simulink model "a_ASXX_MWIN_FLW_filupxxxxg_A"  (R2016b)
settings: Solver=FixedStepDiscrete  StartTime=0.0  StopTime=1  RelTol=1e-3  EnableMultiTasking=on
values from neighbouring files (symbols this model uses):
  Cbx_cyl_fill_efy_intk_mfld_prs_atm_prs_cor_cho = true    [Calib_mdl_RSA.m]
  Cbx_cyl_fill_efy_opt_cho = false    [Calib_mdl_RSA.m]
  Cbx_cyl_fill_igr_opt_cho = false    [Calib_mdl_RSA.m]
  Cnx_cyl_fill_ex_mfld_prs_cor_cho = 0    [Cal_basic.m]
  Cnx_cyl_nr_conf = 3    [Cal_basic.m]
  Cxx_cyl_fill_efy_drv_max = 20    [Calib_mdl_RSA.m]
  Cxx_cyl_fill_efy_dyn_max = 0.15    [Calib_mdl_RSA.m]
  Cxx_cyl_fill_efy_dyn_min = 0    [Calib_mdl_RSA.m]
  Cxx_cyl_fill_efy_dz = 0.45    [Calib_mdl_RSA.m]
  Cxx_cyl_fill_efy_vvt_ofs = 0    [Calib_mdl_RSA.m]
  Cxx_cyl_fill_trap_area_h_thd = 0.2    [Cal_basic.m]
  Cxx_cyl_fill_trap_area_l_thd = 0.1    [Cal_basic.m]
  Cxx_cyl_fill_trap_efy_dz_l_thd = 1    [Cal_basic.m]
  Cxx_cyl_fill_trap_efy_dz_neg_slop = -0.5    [Cal_basic.m]
  Cxx_cyl_fill_trap_efy_dz_pos_slop = 0.5    [Cal_basic.m]
  Cxx_cyl_vol = 3.9961e-04*3    (= 0.00119883)    [Cal_basic.m]    (also in Calib_mdl_RSA.m = 0.00119900004938)
  Cxx_min_cyl_fill_mdl_ex_mfld_prs_rat_cor = 0    [Cal_basic.m]
  Nnx_eng_run_stt = 2    [Calib_mdl_RSA.m]
  Nxx_atm_kpa = 101.3    [Cal_basic.m]
  Nxx_k_degc = 273.15    [Cal_basic.m]
  Nxx_kilo_bas = 1000    [Cal_basic.m]
  Nxx_wht_pgc_j_kg = 287    [Cal_basic.m]
undefined symbols (not defined in the file or in its folder): docblock
libraries: AEMS_Standard_Library x63, simulink x1
(part 1 of 3)
Description:
  | TITLE: Calculation of the volumetric efficiency correction
  | Object of the element: This document specifies the calculation of the cylinder fill-up efficiency depending on pressure, engine speed,VVT angle and VVL position.
settings Model: Creator=z005139  LastModifiedBy=a002701
settings Model: ModifiedHistory=|
  | <Delivery_cycle>: MD13
  | <Author>: f046779
  | <Revision>: 7-0
  | <Nature_of_modifications>: <IS130624>: AEMS / EAL computational problem during a smooth start HR12DDV
  | <Nature_of_modifications>: <IS130784>: AEMS / Wrong calculation of trapping efficiency
  | <Nature_of_modifications>: <IS130844>: AEMS / Insufficient air filling correction in altitude
  | 
  | <Delivery_cycle>: MD12
  | <Author>: p080490
  | <Revision>: 6-0
  | <Nature_of_modifications>: <IS129656>: AEMS / Estimated trapping efficiency impact on exhaust richness setpoint
  | 
  | <Delivery_cycle>: MD11
  | <Author>: p097653
  | <Revision>: 5-0
  | <Nature_of_modifications>: <CR010224>: [IS][AEMS Step2] Issue correction for AE MD11 modules
  | <Nature_of_modifications>: <CR009896>: [AEMS Step2][LPG][Archi] Legacy Migration pour MD11
  | <Nature_of_modifications>: <IS128079>: AEMS / Wrong air filling model correction with atmospheric pressure and deltaP_GPF
  | 
  | <Delivery_cycle>: MD10
  | <Author>: a002701
  | <Revision>: 4-0
  | <Nature_of_modifications>: <CR009236>: [AEMS Step1.9][Gasoline] Update of Engine model improvement (part2)
  | 
  | <Delivery_cycle>: MD09
  | <Author>: p095922
  | <Revision>: 3-0
  | <Nature_of_modifications>: <CR009534>: [IS][A-EMS] Issue correction for AE MD09 modules
  | <Nature_of_modifications>: <IS124783>: AEMS /Wrong constant (Nxx_atm_hpa) used for atmospheric pressure (kpa) related calculation
  | <Nature_of_modifications>: <IS124785>: AEMS /Wrong IGR mass caculation of air filling model
  | 
  | <Delivery_cycle>: MD08
  | <Author>: a002701
  | <Revision>: 2-0
  | <Nature_of_modifications>: <CR006368> : [A-ems step2]  [EFE] Engine model improvement
  | <Nature_of_modifications>: <CR006372>: VVT drift learning usage
  | 
  | <Delivery_cycle>: MD07.02
  | <Author>: p095922
  | <Revision>: 1-0
  | <Nature_of_modifications>: <CR006362>: [A-ems step2] [SUPAS] Intake manifold & boost pressure setpoint
  | <Nature_of_modifications>: <CR008239>: Engine filling & Air flow sensor management
  | <Nature_of_modifications>: <IS122176>: AEMS /[MDL] Underflow occurs for the Output variable Vxx_fill_efv_fuel_rat_raw_20ms
  | 
  | <Delivery_cycle>: MD06.02
  | <Author>: p092015
  | <Revision>: 0-0
  | <Nature_of_modifications>: <CR007978>: [AEMS Step1.9] [Gasoline] GE-R migration
  | 
  | <Delivery_cycle>: LM55_01
  | <Author>: Vuong-son LUONG
  | <Revision>: Rev 35.0
  | <Nature_of_modifications>: <CR007978>: [AEMS Step1.9] [Gasoline] GE-R migration (DMFI04672: [WAMA]: Needed dictionary update for LM55)
  | 
  | <Delivery_cycle>: LM52_01
  | <Author>: Rodolphe BOU TAYEH
  | <Revision>: Rev 34.0
  | <Nature_of_modifications>: <CR007978>: [AEMS Step1.9] [Gasoline] GE-R migration (DMFI04008[LPG] New labels for a specific LPG tuning - Torque management)
  | 
  | <Delivery_cycle>: LM50_01
  | <Author>: Bada NDOYE
  | <Revision>: Rev 33.0
  | <Nature_of_modifications>: <CR007978>: [AEMS Step1.9] [Gasoline] GE-R migration (DMFI03942: [MXAM] : MXAM rules update for LM50)
  | <Nature_of_modifications>: <CR007978>: [AEMS Step1.9] [Gasoline] GE-R migration (DMFI03944 [Tool] Models conversion into slx format for LM50)
  | 
  | <Delivery_cycle>: LM49
  | <Author>: Sarah TALEB
  | <Revision>: Rev 32.0
  | <Nature_of_modifications>: <CR007978>: [AEMS Step1.9] [Gasoline] GE-R migration (DMFI03797 [FLEX] Fill-up correction during transient conditions in Flex Fuel applications)
  | 
  | <Delivery_cycle>: LM47_01
  | <Author>: R.IRAQI
  | <Revision>: Rev 31.0
  | <Nature_of_modifications>: <CR007978>: [AEMS Step1.9] [Gasoline] GE-R migration (DMFI03552 [MXAM] : MXAM rules update for LM47)
  | <Nature_of_modifications>: <CR007978>: [AEMS Step1.9] [Gasoline] GE-R migration (DMFI03553: [WAMA]: Needed dictionary update for LM47)
  | 
  | <Delivery_cycle>: LM42_01
  | <Author>: Hugo DAMANCE
  | <Revision>: Rev 30.0
  | <Nature_of_modifications>: <CR007978>: [AEMS Step1.9] [Gasoline] GE-R migration (DMFI02878 [MXAM] : MXAM rules update for LM42)
  | 
  | <Delivery_cycle>: LM41_01
  | <Author>: Antoine NAIIM HABIB
  | <Revision>: Rev 29.0
  | <Nature_of_modifications>: <CR007978>: [AEMS Step1.9] [Gasoline] GE-R migration (ISMET27009 K3: [SPEC] Wrong use of Interp library with shared axis in IN_ASI_IAF_2)
  | <Nature_of_modifications>: <CR007978>: [AEMS Step1.9] [Gasoline] GE-R migration (DMFI02746: [Floating] Actual integer data typing to reach one click auto-coding)
  | <Nature_of_modifications>: <CR007978>: [AEMS Step1.9] [Gasoline] GE-R migration (ISMET29395 K4: [SPEC] Evolution of range for coherency in a_in_asi_iaf_filupxx_xxx_xx_g_a)
  | 
  | <Delivery_cycle>: AEG_39_01
  | <Author>: Cheng-Qiang HE
  | <Revision>: Rev 28.0
  | <Nature_of_modifications>: <CR007978>: [AEMS Step1.9] [Gasoline] GE-R migration (ISSUP21633 K3: Issue in model La table Ctp_fill_efy_cor_dyn_amp_rat ne doit pas avoir d'axes partages)
  | <Nature_of_modifications>: <CR007978>: [AEMS Step1.9] [Gasoline] GE-R migration (DMFI02368: [Floating] Modification of specification to comply with floating autocoding LM39)
  | 
  | <Delivery_cycle>: AEG_34_01
  | <Author>: YOBOUE Konan
  | <Revision>: Rev 27.0
  | <Nature_of_modifications>: <CR007978>: [AEMS Step1.9] [Gasoline] GE-R migration (IS19506 (K2): Ctb_mat2 is not anymore referenced by InAsiIat)
  | 
  | <Delivery_cycle>: LM_XX
  | <Author>: KIEFFER Steve
  | <Revision>: Rev 26.0
  | <Nature_of_modifications>: <CR007978>: [AEMS Step1.9] [Gasoline] GE-R migration (ISMAP18189 : Altitude correction for fill-up model)
  | 
  | <Delivery_cycle>: LM_XX
  | <Author>: KIEFFER Steve
  | <Revision>: Rev 25.0
  | <Nature_of_modifications>: <CR007978>: [AEMS Step1.9] [Gasoline] GE-R migration (ISSUP K2 13588 : Breakpoints shall be given under referenced section in MID)
  | <Nature_of_modifications>: <CR007978>: [AEMS Step1.9] [Gasoline] GE-R migration (ISMAP K3 15074 : Range correction of cmp_n_map_fill_efv_ofs_alco)
  | 
  | <Delivery_cycle>: LM_XX
  | <Author>: THOUVENEL Nicolas
  | <Revision>: Rev 24.0
  | <Nature_of_modifications>: <CR007978>: [AEMS Step1.9] [Gasoline] GE-R migration (ISMET13261 : Modification for dynamic fill-up efficiency computation)
  | 
  | <Delivery_cycle>: LM_XX
  | <Author>: THOUVENEL Nicolas
  | <Revision>: Rev 23.0
  | <Nature_of_modifications>: <CR007978>: [AEMS Step1.9] [Gasoline] GE-R migration (ISMAP 11648 : Dynamic Over fill-up)
  | <Nature_of_modifications>: <CR007978>: [AEMS Step1.9] [Gasoline] GE-R migration (ISMET 12293 : Taking into account of injected fuel flow drift function as Tcarb over F4Rt87x)
  | <Nature_of_modifications>: <CR007978>: [AEMS Step1.9] [Gasoline] GE-R migration (ISMET 12394 : Dictionary to be modified for dissociating variables Vxx_fill_efy_cor_dyn_amp_raw &amp; Vxx_fill_efy_cor_dyn_raw)
  | <Nature_of_modifications>: <CR007978>: [AEMS Step1.9] [Gasoline] GE-R migration (ISMAP 12637 : Basic tuning impossible with ASG_26 (implementation of cylinder deactivation)
  | <Nature_of_modifications>: <CR007978>: [AEMS Step1.9] [Gasoline] GE-R migration (ISMET 12912 : Modification of logical naming for cartography of cylinder deactivation)
  | 
  | <Delivery_cycle>: LM_XX
  | <Author>: BANZET Sebastien
  | <Revision>: Rev 22.0
  | <Nature_of_modifications>: <CR007978>: [AEMS Step1.9] [Gasoline] GE-R migration (DMFI Amont 207 : Cylinder deactivation)
  | <Nature_of_modifications>: <CR007978>: [AEMS Step1.9] [Gasoline] GE-R migration (DMFI 833 : [Flex/Gasoline] : Separated management for Flex &amp; Gasoline tuning values #2)
  | <Nature_of_modifications>: <CR007978>: [AEMS Step1.9] [Gasoline] GE-R migration (ISMET 10136 : implementation of intermediate variables for fill-up efficiency calculation)
  | <Nature_of_modifications>: <CR007978>: [AEMS Step1.9] [Gasoline] GE-R migration (ISMET 10468 : Check revision of timer block)
  | 
  | <Delivery_cycle>: LM_XX
  | <Author>: THOUVENEL Nicolas
  | <Revision>: Rev 21.0
  | <Nature_of_modifications>: <CR007978>: [AEMS Step1.9] [Gasoline] GE-R migration (ISMET 09504 : Fill-up and Trapping models correction with taking into account atmospheric pressure)
  | 
  | <Delivery_cycle>: LM_XX
  | <Author>: HEBERT
  | <Revision>: Rev 20.0
  | <Nature_of_modifications>: <CR007978>: [AEMS Step1.9] [Gasoline] GE-R migration (ISMET05853: Modification of Vxx_vvt_fill_efv_cor_fac1 range and resol. Correction of Cmp_vvt_fill_efv_cor_fac1 bounds) (a_in_asi_iaf_filupxx_xxx_xx_g_a)
  | 
  | <Delivery_cycle>: LM_XX
  | <Author>: THOUVENEL
  | <Revision>: Rev 19.3
  | <Nature_of_modifications>: <CR007978>: [AEMS Step1.9] [Gasoline] GE-R migration (Update to ISMET 05742) (a_in_asi_iaf_filupxx_xxx_xx_g_a)
  | 
  | <Delivery_cycle>: LM_XX
  | <Author>: THOUVENEL
  | <Revision>: Rev 19.2
  | <Nature_of_modifications>: <CR007978>: [AEMS Step1.9] [Gasoline] GE-R migration (Correction of resolution of Vxx_fill_efy_cor_dyn) (a_in_asi_iaf_filupxx_xxx_xx_g_a)
  | 
  | <Delivery_cycle>: LM_XX
  | <Author>: THOUVENEL
  | <Revision>: Rev 19.1
  | <Nature_of_modifications>: <CR007978>: [AEMS Step1.9] [Gasoline] GE-R migration (IS 04502 : "Missing documentation in a_in_asi_iaf_filupxx_xxx_xx_g_a(19.0)") (a_in_asi_iaf_filupxx_xxx_xx_g_a)
  | 
  | <Delivery_cycle>: LM_XX
  | <Author>: THOUVENEL
  | <Revision>: Rev 19.0
  | <Nature_of_modifications>: <CR007978>: [AEMS Step1.9] [Gasoline] GE-R migration (Implementation of volumetric correction for Dual VVT (intake, exhaust)) (a_in_asi_iaf_filupxx_xxx_xx_g_a)
  | 
  | <Delivery_cycle>: LM_XX
  | <Author>: LENOIR
  | <Revision>: Rev 18.0
  | <Nature_of_modifications>: <CR007978>: [AEMS Step1.9] [Gasoline] GE-R migration (ISMAP_2163: Add New calibration Cmp_n_map_cor_dyn_amp, Ctp_fill_efy_cor_dyn_amp_rat, Ctb_fill_efy_cor_dyn_amp, New Input Vxx_amp, Change resolution of Cmp_n_map_cor_dyn_th) (a_in_asi_iaf_filupxx_xxx_xx_g_a)
  | 
  | <Delivery_cycle>: LM_XX
  | <Author>: LENOIR
  | <Revision>: Rev 17.0
  | <Nature_of_modifications>: <CR007978>: [AEMS Step1.9] [Gasoline] GE-R migration (IS_MAP 420 :  Add the "thermic" factor to correct the fill-up efficiency (figure 4) =&gt; New Inputs : Vsx_eng, Vxx_tco=&gt; New internal variables :Vxx_fill_efy_cor_dyn, Vxx_fill_efy_cor_dyn_raw.=&gt; New calibrations : Cmp_n_map_cor_dyn_th, Ctb_n_fill_efy_cor_dyn, Ctb_tco2, Ctp_map_n_ftc,  Cxx_fill_efy_cor_dyn_max, Cxx_fill_efy_cor_dyn_min,  Nsx_eng_aut) (a_in_asi_iaf_filupxx_xxx_xx_g_a)
  | 
  | <Delivery_cycle>: LM_XX
  | <Author>: WALRAVE
  | <Revision>: Rev 16.0
  | <Nature_of_modifications>: <CR007978>: [AEMS Step1.9] [Gasoline] GE-R migration (reopening of ISMAP 32 : Resolutions of Cmp_vvt_fill_efv_cor_fac1, Cmp_vvt_fill_efv_cor_fac2, Vxx_vvt_fill_efv_cor_fac1, Vxx_vvt_fill_efv_cor_fac2 has been divided by 256. ranges unchanged) (a_in_asi_iaf_filupxx_xxx_xx_g_a)
  | 
  | <Delivery_cycle>: LM_XX
  | <Author>: WALRAVE
  | <Revision>: Rev 15.0
  | <Nature_of_modifications>: <CR007978>: [AEMS Step1.9] [Gasoline] GE-R migration (Alcool settings added offset of fill up efficiency coming form alcoxxx spec as well as specific temperature correction for alcool LPG removed new document model) (a_in_asi_iaf_filupxx_xxx_xx_g_a)
  | 
  | <Delivery_cycle>: LM_XX
  | <Author>: WALRAVE
  | <Revision>: Rev 14.0
  | <Nature_of_modifications>: <CR007978>: [AEMS Step1.9] [Gasoline] GE-R migration (Bug correction on VVT parameter. Cmp_vvt_fill_efv_cor_fac1 and fac2 have a new resolution and range. As well as Vxx_vvt_fill_efv_cor_fac1 and fac2. Bloc names changed to respect rules) (a_in_asi_iaf_filupxx_xxx_xx_g_a)
  | 
  | <Delivery_cycle>: LM_XX
  | <Author>: ALLACH
  | <Revision>: Rev 13.0
  | <Nature_of_modifications>: <CR007978>: [AEMS Step1.9] [Gasoline] GE-R migration (Add Shared index Vxb_n in Cmp_vvt_fill_efv_cor_fac1 Cmp_vvt_fill_efv_cor_fac2 Cmp_n_map_fill_efv Cmp_n_map_fill_efv_lpg RSA_BKPT_2D block) (a_in_asi_iaf_filupxx_xxx_xx_g_a)
  | 
  | <Delivery_cycle>: LM_XX
  | <Author>: WALRAVE
  | <Revision>: Rev 12.0
  | <Nature_of_modifications>: <CR007978>: [AEMS Step1.9] [Gasoline] GE-R migration (Engine speed IVLD removed. VVT IVLD removed. Slew rate is now before the deadzone on filtered fill-up efficiency. Comments corrected) (a_in_asi_iaf_filupxx_xxx_xx_g_a)
  | 
  | <Delivery_cycle>: LM_XX
  | <Author>: WALRAVE
  | <Revision>: Rev 11.0
  | <Nature_of_modifications>: <CR007978>: [AEMS Step1.9] [Gasoline] GE-R migration (Update of the IVLD construction. Added init values. Removed replacement values for inputs Document model modified) (a_in_asi_iaf_filupxx_xxx_xx_g_a)
  | 
  | <Delivery_cycle>: LM_XX
  | <Author>: WALRAVE
  | <Revision>: Rev 10.0
  | <Nature_of_modifications>: <CR007978>: [AEMS Step1.9] [Gasoline] GE-R migration (Modification for IS 109 : Library blocks are used instead in the filter block for the throttle command) (a_in_asi_iaf_filupxx_xxx_xx_g_a)
  | 
  | <Delivery_cycle>: LM_XX
  | <Author>: WALRAVE
  | <Revision>: Rev 9.0
  | <Nature_of_modifications>: <CR007978>: [AEMS Step1.9] [Gasoline] GE-R migration (strategy for ON/OFF VVT removed. Vbx_vvt_cart_ti removed) (a_in_asi_iaf_filupxx_xxx_xx_g_a)
  | 
  | <Delivery_cycle>: LM_XX
  | <Author>: WALRAVE
  | <Revision>: Rev 8.0
  | <Nature_of_modifications>: <CR007978>: [AEMS Step1.9] [Gasoline] GE-R migration (Coherency done. vvt variables changed into standard types) (a_in_asi_iaf_filupxx_xxx_xx_g_a)
  | 
  | <Delivery_cycle>: LM_XX
  | <Author>: WALRAVE
  | <Revision>: Rev 7.0
  | <Nature_of_modifications>: <CR007978>: [AEMS Step1.9] [Gasoline] GE-R migration (New output Vxx_eng_vol_fill_efy_fil created for throttle command. Deadzone filter + rate limiter) (a_in_asi_iaf_filupxx_xxx_xx_g_a)
  | 
  | <Delivery_cycle>: LM_XX
  | <Author>: WALRAVE
  | <Revision>: Rev 6.0
  | <Nature_of_modifications>: <CR007978>: [AEMS Step1.9] [Gasoline] GE-R migration (RSI on RD8_020: Vxx_vvt_fill_efv_cor_fac2 range, resol and unit modified. Cmp_vvt_fill_efv_cor_fac2 range, resol &amp; unit modified. Several units corrected to be more explicit and standard) (a_in_asi_iaf_filupxx_xxx_xx_g_a)
  | 
  | <Delivery_cycle>: LM_XX
  | <Author>: PORCHEROT
  | <Revision>: Rev 5.0
  | <Nature_of_modifications>: <CR007978>: [AEMS Step1.9] [Gasoline] GE-R migration (Comment and state changed for Vsx_n_vld) (a_in_asi_iaf_filupxx_xxx_xx_g_a)
  | 
  | <Delivery_cycle>: LM_XX
  | <Author>: WALRAVE
  | <Revision>: Rev 4.0
  | <Nature_of_modifications>: <CR007978>: [AEMS Step1.9] [Gasoline] GE-R migration (Bloc "Validity_indicator" modified (two NOT added). Correction of Ctb_mat2 (input variable)) (a_in_asi_iaf_filupxx_xxx_xx_g_a)
  | 
  | <Delivery_cycle>: LM_XX
  | <Author>: WALRAVE
  | <Revision>: Rev 3.0
  | <Nature_of_modifications>: <CR007978>: [AEMS Step1.9] [Gasoline] GE-R migration (Validity indicators added. Correction for RSI 63 : resolution of Cmp_vvt_fill_efv_cor_fac1 modified) (a_in_asi_iaf_filupxx_xxx_xx_g_a)
  | 
  | <Delivery_cycle>: LM_XX
  | <Author>: ADMIN
  | <Revision>: Rev 2.1
  | <Nature_of_modifications>: <CR007978>: [AEMS Step1.9] [Gasoline] GE-R migration (Ctb_prs ( New max = 20000]), Vxx_in_vvtc_angl ( New max = 96[ New unit = DegCrk), Vxx_map ( New max = 20000])) (a_in_asi_iaf_filupxx_xxx_xx_g_a)
  | 
  | <Delivery_cycle>: LM_XX
  | <Author>: WALRAVE
  | <Revision>: Rev 2.0
  | <Nature_of_modifications>: <CR007978>: [AEMS Step1.9] [Gasoline] GE-R migration (Dictionary update + cartography dimension changed) (a_in_asi_iaf_filupxx_xxx_xx_g_a)
  | 
  | <Delivery_cycle>: LM_XX
  | <Author>: WALRAVE
  | <Revision>: Rev 1.1
  | <Nature_of_modifications>: <CR007978>: [AEMS Step1.9] [Gasoline] GE-R migration (Range &amp; resol corrected) (a_in_asi_iaf_filupxx_xxx_xx_g_a)
  | 
  | <Delivery_cycle>: LM_XX
  | <Author>: WALRAVE
  | <Revision>: Rev 1.0
  | <Nature_of_modifications>: <CR007978>: [AEMS Step1.9] [Gasoline] GE-R migration (Fillup efficiency is now physical (ratio near 1).It includes the effect of temperature that was in a_im_airxx_a5_a) (a_in_asi_iaf_filupxx_xxx_xx_g_a)
settings DataIOCC: SaveFormat=StructureWithTime
settings OptimizationCC: DefaultUnderspecifiedDataType=single  LifeSpan=inf
settings DebuggingCC: SignalInfNanChecking=error  SignalRangeChecking=error  AlgebraicLoopMsg=error  ArtificialAlgebraicLoopMsg=error  SaveWithParameterizedLinksMsg=error  CheckSSInitialOutputMsg=off  BlockPriorityViolationMsg=error  MinStepSizeMsg=error  SolverPrmCheckMsg=warning  InheritedTsInSrcMsg=error  TasksWithSamePriorityMsg=error  SigSpecEnsureSampleTimeMsg=error  CheckMatrixSingularityMsg=error  IntegerOverflowMsg=error  ParameterUnderflowMsg=error  ParameterPrecisionLossMsg=none  ParameterTunabilityLossMsg=error  FixptConstUnderflowMsg=error  FixptConstOverflowMsg=error  FixptConstPrecisionLossMsg=error  UnderSpecifiedDataTypeMsg=warning  UnnecessaryDatatypeConvMsg=warning  SignalLabelMismatchMsg=warning  UnconnectedInputMsg=error  UnconnectedOutputMsg=error  UnconnectedLineMsg=error  SFcnCompatibilityMsg=error  FrameProcessingCompatibilityMsg=warning  BusObjectLabelMismatch=error  RootOutportRequireBusObject=error  AllowSymbolicDim=off  ModelReferenceIOMsg=warning  ModelReferenceIOMismatchMessage=error  UnknownTsInhSupMsg=error  ModelReferenceDataLoggingMessage=error  StateNameClashWarn=warning  SimStateInterfaceChecksumMismatchMsg=error  StrictBusMsg=ErrorOnBusTreatedAsVector  NonBusSignalsTreatedAsBus=error  SFUnusedDataAndEventsDiag=error  SFInvalidInputDataAccessInChartInitDiag=error  SFTransitionOutsideNaturalParentDiag=error  SFUnreachableExecutionPathDiag=error  SFUndirectedBroadcastEventsDiag=error  SFOutputUsedAsStateInMooreChartDiag=none  SFTemporalDelaySmallerThanSampleTimeDiag=none  SFSelfTransitionDiag=error  SFExecutionAtInitializationDiag=none  UnitsInconsistencyMsg=none  AllowAutomaticUnitConversions=off
settings HardwareCC: ProdBitPerPointer=32  ProdBitPerSizeT=32  ProdBitPerPtrDiffT=32  ProdLargestAtomicInteger=Integer  ProdLargestAtomicFloat=None  ProdIntDivRoundTo=Undefined  ProdEndianess=Unspecified  ProdWordSize=32  ProdHWDeviceType=32-bit Generic
settings ModelReferenceCC: UpdateModelReferenceTargets=IfOutOfDate  EnableParallelModelReferenceBuilds=on  ParallelModelReferenceErrorOnInvalidPool=off  ModelReferenceNumInstancesAllowed=Single  PropagateSignalLabelsOutOfModel=off
settings SFSimCC: SFSimEcho=off  SimGenImportedTypeDefs=on
settings RTWCC: GenerateMakefile=off
settings GRTTargetCC: CodeReplacementLibrary=ANSI_C  MatFileLogging=off
settings ConfigComp: CovMetricSettings=dcmtrzoibsw  CovHtmlReporting=on  CovSaveCumulativeToWorkspaceVar=on  CovSaveSingleToWorkspaceVar=on  CovCumulativeReport=on

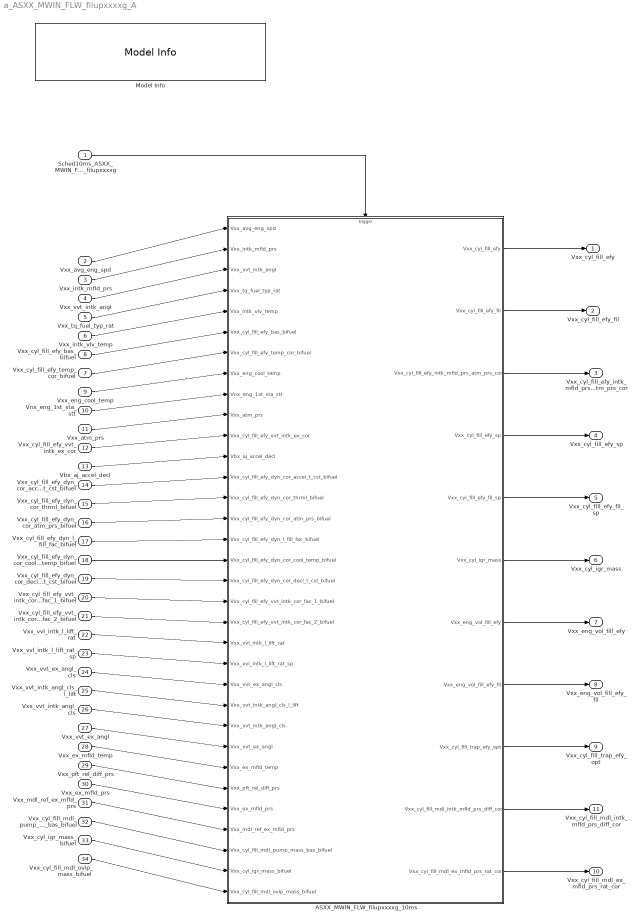
== system a_ASXX_MWIN_FLW_filupxxxxg_A ==
  Sched10ms_ASXX_MWIN_FLW_filupxxxxg : Inport  Interpolate=off  OutputFunctionCall=on
  Vxx_avg_eng_spd : Inport  Port=2  Interpolate=off
  Vxx_intk_mfld_prs : Inport  Port=3  Interpolate=off
  Vxx_vvt_intk_angl : Inport  Port=4  Interpolate=off
  Vxx_tq_fuel_typ_rat : Inport  Port=5  Interpolate=off
  Vxx_intk_vlv_temp : Inport  Port=6  Interpolate=off
  Vxx_cyl_fill_efy_temp_cor_bifuel : Inport  Port=7  Interpolate=off
  Vxx_cyl_fill_efy_bas_bifuel : Inport  Port=8  Interpolate=off
  Vxx_eng_cool_temp : Inport  Port=9  Interpolate=off
  Vnx_eng_1st_sta_stt : Inport  Port=10  Interpolate=off
  Vxx_atm_prs : Inport  Port=11  Interpolate=off
  Vxx_cyl_fill_efy_vvt_intk_ex_cor : Inport  Port=12  Interpolate=off
  Vbx_aj_accel_decl : Inport  Port=13  Interpolate=off
  Vxx_cyl_fill_efy_dyn_cor_accel_t_cst_bifuel : Inport  Port=14  Interpolate=off
  Vxx_cyl_fill_efy_dyn_cor_thrml_bifuel : Inport  Port=15  Interpolate=off
  Vxx_cyl_fill_efy_dyn_cor_atm_prs_bifuel : Inport  Port=16  Interpolate=off
  Vxx_cyl_fill_efy_dyn_l_fill_fac_bifuel : Inport  Port=17  Interpolate=off
  Vxx_cyl_fill_efy_dyn_cor_cool_temp_bifuel : Inport  Port=18  Interpolate=off
  Vxx_cyl_fill_efy_dyn_cor_decl_t_cst_bifuel : Inport  Port=19  Interpolate=off
  Vxx_cyl_fill_efy_vvt_intk_cor_fac_1_bifuel : Inport  Port=20  Interpolate=off
  Vxx_cyl_fill_efy_vvt_intk_cor_fac_2_bifuel : Inport  Port=21  Interpolate=off
  Vxx_vvl_intk_l_lift_rat : Inport  Port=22  Interpolate=off
  Vxx_vvl_intk_l_lift_rat_sp : Inport  Port=23  Interpolate=off
  Vxx_vvt_ex_angl_cls : Inport  Port=24  Interpolate=off
  Vxx_vvt_intk_angl_cls_l_lift : Inport  Port=25  Interpolate=off
  Vxx_vvt_intk_angl_cls : Inport  Port=26  Interpolate=off
  Vxx_vvt_ex_angl : Inport  Port=27  Interpolate=off
  Vxx_ex_mfld_temp : Inport  Port=28  Interpolate=off
  Vxx_pft_rel_diff_prs : Inport  Port=29  Interpolate=off
  Vxx_ex_mfld_prs : Inport  Port=30  Interpolate=off
  Vxx_mdl_ref_ex_mfld_prs : Inport  Port=31  Interpolate=off
  Vxx_cyl_fill_mdl_pump_mass_bas_bifuel : Inport  Port=32  Interpolate=off
  Vxx_cyl_igr_mass_bifuel : Inport  Port=33  Interpolate=off
  Vxx_cyl_fill_mdl_ovlp_mass_bifuel : Inport  Port=34  Interpolate=off
  ASXX_MWIN_FLW_filupxxxxg_10ms : Subsystem  Tag=[RUNNABLE]  TreatAsAtomicUnit=on  RTWFileName=InAsiIaf_Filupxx_xxxxxg
      settings: AttributesFormatString=%<Tag>  RTWSystemCode=Nonreusable function  RTWFcnNameOpts=Use subsystem name  RTWFileNameOpts=User specified
  Model Info : simulink/Model-Wide Utilities/Model Info  Frame=on  DisplayStringWithTags=|  HorizontalTextAlignment=Center  LeftAlignmentValue=0.5  SourceBlockDiagram=a_ASXX_MWIN_FLW_filupxxxxg_A  TagMaxNumber=20
      | Model Info
      | %<ModelVersion>
      | Editor: %<LastModifiedBy>
      | Last modified: %<LastModificationDate>
  Vxx_cyl_fill_efy : Outport
  Vxx_cyl_fill_efy_fil : Outport  Port=2
  Vxx_cyl_fill_efy_intk_mfld_prs_atm_prs_cor : Outport  Port=3
  Vxx_cyl_fill_efy_sp : Outport  Port=4
  Vxx_cyl_fill_efy_fil_sp : Outport  Port=5
  Vxx_cyl_igr_mass : Outport  Port=6
  Vxx_eng_vol_fill_efy : Outport  Port=7
  Vxx_eng_vol_fill_efy_fil : Outport  Port=8
  Vxx_cyl_fill_trap_efy_opt : Outport  Port=9
  Vxx_cyl_fill_mdl_ex_mfld_prs_rat_cor : Outport  Port=10
  Vxx_cyl_fill_mdl_intk_mfld_prs_diff_cor : Outport  Port=11
  wires:
  Vxx_cyl_fill_efy_vvt_intk_cor_fac_2_bifuel/1 -> ASXX_MWIN_FLW_filupxxxxg_10ms/20(Vxx_cyl_fill_efy_vvt_intk_cor_fac_2_bifuel)
  Vxx_cyl_fill_efy_vvt_intk_cor_fac_1_bifuel/1 -> ASXX_MWIN_FLW_filupxxxxg_10ms/19(Vxx_cyl_fill_efy_vvt_intk_cor_fac_1_bifuel)
  Vxx_cyl_fill_efy_dyn_cor_decl_t_cst_bifuel/1 -> ASXX_MWIN_FLW_filupxxxxg_10ms/18(Vxx_cyl_fill_efy_dyn_cor_decl_t_cst_bifuel)
  Vxx_cyl_fill_efy_dyn_cor_cool_temp_bifuel/1 -> ASXX_MWIN_FLW_filupxxxxg_10ms/17(Vxx_cyl_fill_efy_dyn_cor_cool_temp_bifuel)
  Vxx_cyl_fill_efy_dyn_l_fill_fac_bifuel/1 -> ASXX_MWIN_FLW_filupxxxxg_10ms/16(Vxx_cyl_fill_efy_dyn_l_fill_fac_bifuel)
  Vxx_cyl_fill_efy_dyn_cor_atm_prs_bifuel/1 -> ASXX_MWIN_FLW_filupxxxxg_10ms/15(Vxx_cyl_fill_efy_dyn_cor_atm_prs_bifuel)
  Vxx_cyl_fill_efy_dyn_cor_thrml_bifuel/1 -> ASXX_MWIN_FLW_filupxxxxg_10ms/14(Vxx_cyl_fill_efy_dyn_cor_thrml_bifuel)
  Vxx_cyl_fill_efy_dyn_cor_accel_t_cst_bifuel/1 -> ASXX_MWIN_FLW_filupxxxxg_10ms/13(Vxx_cyl_fill_efy_dyn_cor_accel_t_cst_bifuel)
  Vxx_avg_eng_spd/1 -> ASXX_MWIN_FLW_filupxxxxg_10ms/1(Vxx_avg_eng_spd)
  Vxx_intk_mfld_prs/1 -> ASXX_MWIN_FLW_filupxxxxg_10ms/2(Vxx_intk_mfld_prs)
  Vxx_vvt_intk_angl/1 -> ASXX_MWIN_FLW_filupxxxxg_10ms/3(Vxx_vvt_intk_angl)
  Vxx_tq_fuel_typ_rat/1 -> ASXX_MWIN_FLW_filupxxxxg_10ms/4(Vxx_tq_fuel_typ_rat)
  Vxx_intk_vlv_temp/1 -> ASXX_MWIN_FLW_filupxxxxg_10ms/5(Vxx_intk_vlv_temp)
  Sched10ms_ASXX_MWIN_FLW_filupxxxxg/1 -> ASXX_MWIN_FLW_filupxxxxg_10ms/Trigger
  Vxx_cyl_fill_efy_temp_cor_bifuel/1 -> ASXX_MWIN_FLW_filupxxxxg_10ms/7(Vxx_cyl_fill_efy_temp_cor_bifuel)
  Vxx_cyl_fill_efy_bas_bifuel/1 -> ASXX_MWIN_FLW_filupxxxxg_10ms/6(Vxx_cyl_fill_efy_bas_bifuel)
  Vxx_eng_cool_temp/1 -> ASXX_MWIN_FLW_filupxxxxg_10ms/8(Vxx_eng_cool_temp)
  Vnx_eng_1st_sta_stt/1 -> ASXX_MWIN_FLW_filupxxxxg_10ms/9(Vnx_eng_1st_sta_stt)
  Vxx_atm_prs/1 -> ASXX_MWIN_FLW_filupxxxxg_10ms/10(Vxx_atm_prs)
  Vxx_cyl_fill_efy_vvt_intk_ex_cor/1 -> ASXX_MWIN_FLW_filupxxxxg_10ms/11(Vxx_cyl_fill_efy_vvt_intk_ex_cor)
  Vbx_aj_accel_decl/1 -> ASXX_MWIN_FLW_filupxxxxg_10ms/12(Vbx_aj_accel_decl)
  ASXX_MWIN_FLW_filupxxxxg_10ms/1(Vxx_cyl_fill_efy) -> Vxx_cyl_fill_efy/1
  ASXX_MWIN_FLW_filupxxxxg_10ms/2(Vxx_cyl_fill_efy_fil) -> Vxx_cyl_fill_efy_fil/1
  ASXX_MWIN_FLW_filupxxxxg_10ms/3(Vxx_cyl_fill_efy_intk_mfld_prs_atm_prs_cor) -> Vxx_cyl_fill_efy_intk_mfld_prs_atm_prs_cor/1
  ASXX_MWIN_FLW_filupxxxxg_10ms/5(Vxx_cyl_fill_efy_fil_sp) -> Vxx_cyl_fill_efy_fil_sp/1
  ASXX_MWIN_FLW_filupxxxxg_10ms/4(Vxx_cyl_fill_efy_sp) -> Vxx_cyl_fill_efy_sp/1
  Vxx_vvl_intk_l_lift_rat/1 -> ASXX_MWIN_FLW_filupxxxxg_10ms/21(Vxx_vvl_intk_l_lift_rat)
  Vxx_vvl_intk_l_lift_rat_sp/1 -> ASXX_MWIN_FLW_filupxxxxg_10ms/22(Vxx_vvl_intk_l_lift_rat_sp)
  Vxx_vvt_ex_angl_cls/1 -> ASXX_MWIN_FLW_filupxxxxg_10ms/23(Vxx_vvt_ex_angl_cls)
  ASXX_MWIN_FLW_filupxxxxg_10ms/6(Vxx_cyl_igr_mass) -> Vxx_cyl_igr_mass/1
  Vxx_vvt_intk_angl_cls/1 -> ASXX_MWIN_FLW_filupxxxxg_10ms/25(Vxx_vvt_intk_angl_cls)
  Vxx_vvt_intk_angl_cls_l_lift/1 -> ASXX_MWIN_FLW_filupxxxxg_10ms/24(Vxx_vvt_intk_angl_cls_l_lift)
  ASXX_MWIN_FLW_filupxxxxg_10ms/7(Vxx_eng_vol_fill_efy) -> Vxx_eng_vol_fill_efy/1
  ASXX_MWIN_FLW_filupxxxxg_10ms/8(Vxx_eng_vol_fill_efy_fil) -> Vxx_eng_vol_fill_efy_fil/1
  ASXX_MWIN_FLW_filupxxxxg_10ms/9(Vxx_cyl_fill_trap_efy_opt) -> Vxx_cyl_fill_trap_efy_opt/1
  Vxx_vvt_ex_angl/1 -> ASXX_MWIN_FLW_filupxxxxg_10ms/26(Vxx_vvt_ex_angl)
  Vxx_ex_mfld_temp/1 -> ASXX_MWIN_FLW_filupxxxxg_10ms/27(Vxx_ex_mfld_temp)
  Vxx_pft_rel_diff_prs/1 -> ASXX_MWIN_FLW_filupxxxxg_10ms/28(Vxx_pft_rel_diff_prs)
  Vxx_ex_mfld_prs/1 -> ASXX_MWIN_FLW_filupxxxxg_10ms/29(Vxx_ex_mfld_prs)
  Vxx_mdl_ref_ex_mfld_prs/1 -> ASXX_MWIN_FLW_filupxxxxg_10ms/30(Vxx_mdl_ref_ex_mfld_prs)
  Vxx_cyl_fill_mdl_pump_mass_bas_bifuel/1 -> ASXX_MWIN_FLW_filupxxxxg_10ms/31(Vxx_cyl_fill_mdl_pump_mass_bas_bifuel)
  Vxx_cyl_igr_mass_bifuel/1 -> ASXX_MWIN_FLW_filupxxxxg_10ms/32(Vxx_cyl_igr_mass_bifuel)
  Vxx_cyl_fill_mdl_ovlp_mass_bifuel/1 -> ASXX_MWIN_FLW_filupxxxxg_10ms/33(Vxx_cyl_fill_mdl_ovlp_mass_bifuel)
  ASXX_MWIN_FLW_filupxxxxg_10ms/11(Vxx_cyl_fill_mdl_ex_mfld_prs_rat_cor) -> Vxx_cyl_fill_mdl_ex_mfld_prs_rat_cor/1
  ASXX_MWIN_FLW_filupxxxxg_10ms/10(Vxx_cyl_fill_mdl_intk_mfld_prs_diff_cor) -> Vxx_cyl_fill_mdl_intk_mfld_prs_diff_cor/1

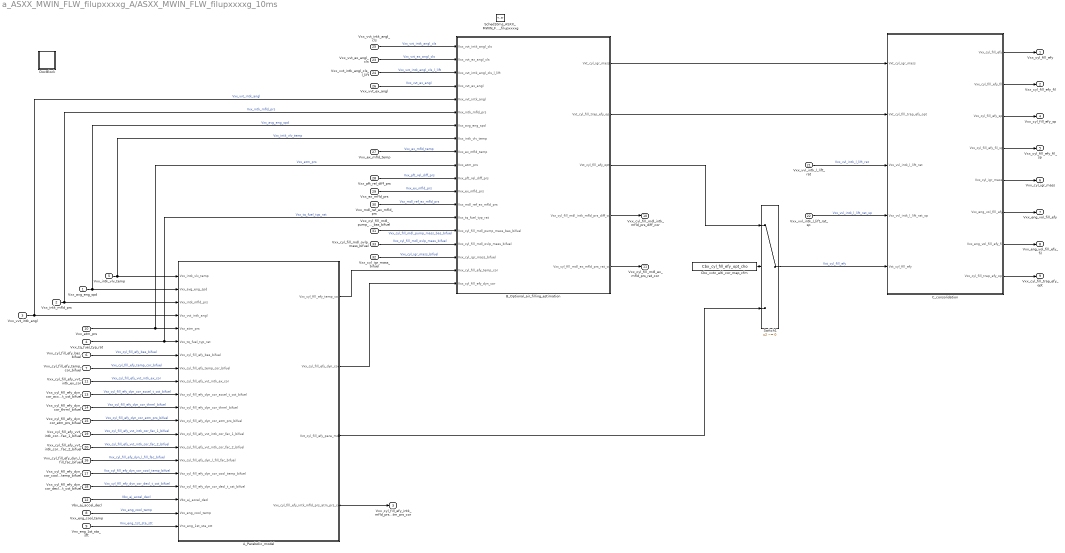
== system a_ASXX_MWIN_FLW_filupxxxxg_A/ASXX_MWIN_FLW_filupxxxxg_10ms ==
  Vxx_avg_eng_spd : Inport  Interpolate=off
  Vxx_intk_mfld_prs : Inport  Port=2  Interpolate=off
  Vxx_vvt_intk_angl : Inport  Port=3  Interpolate=off
  Vxx_tq_fuel_typ_rat : Inport  Port=4  Interpolate=off
  Vxx_intk_vlv_temp : Inport  Port=5  Interpolate=off
  Vxx_cyl_fill_efy_bas_bifuel : Inport  Port=6  Interpolate=off
  Vxx_cyl_fill_efy_temp_cor_bifuel : Inport  Port=7  Interpolate=off
  Vxx_eng_cool_temp : Inport  Port=8  Interpolate=off
  Vnx_eng_1st_sta_stt : Inport  Port=9  Interpolate=off
  Vxx_atm_prs : Inport  Port=10  Interpolate=off
  Vxx_cyl_fill_efy_vvt_intk_ex_cor : Inport  Port=11  Interpolate=off
  Vbx_aj_accel_decl : Inport  Port=12  Interpolate=off
  Vxx_cyl_fill_efy_dyn_cor_accel_t_cst_bifuel : Inport  Port=13  Interpolate=off
  Vxx_cyl_fill_efy_dyn_cor_thrml_bifuel : Inport  Port=14  Interpolate=off
  Vxx_cyl_fill_efy_dyn_cor_atm_prs_bifuel : Inport  Port=15  Interpolate=off
  Vxx_cyl_fill_efy_dyn_l_fill_fac_bifuel : Inport  Port=16  Interpolate=off
  Vxx_cyl_fill_efy_dyn_cor_cool_temp_bifuel : Inport  Port=17  Interpolate=off
  Vxx_cyl_fill_efy_dyn_cor_decl_t_cst_bifuel : Inport  Port=18  Interpolate=off
  Vxx_cyl_fill_efy_vvt_intk_cor_fac_1_bifuel : Inport  Port=19  Interpolate=off
  Vxx_cyl_fill_efy_vvt_intk_cor_fac_2_bifuel : Inport  Port=20  Interpolate=off
  Vxx_vvl_intk_l_lift_rat : Inport  Port=21  Interpolate=off
  Vxx_vvl_intk_l_lift_rat_sp : Inport  Port=22  Interpolate=off
  Vxx_vvt_ex_angl_cls : Inport  Port=23  Interpolate=off
  Vxx_vvt_intk_angl_cls_l_lift : Inport  Port=24  Interpolate=off
  Vxx_vvt_intk_angl_cls : Inport  Port=25  Interpolate=off
  Vxx_vvt_ex_angl : Inport  Port=26  Interpolate=off
  Vxx_ex_mfld_temp : Inport  Port=27  Interpolate=off
  Vxx_pft_rel_diff_prs : Inport  Port=28  Interpolate=off
  Vxx_ex_mfld_prs : Inport  Port=29  Interpolate=off
  Vxx_mdl_ref_ex_mfld_prs : Inport  Port=30  Interpolate=off
  Vxx_cyl_fill_mdl_pump_mass_bas_bifuel : Inport  Port=31  Interpolate=off
  Vxx_cyl_igr_mass_bifuel : Inport  Port=32  Interpolate=off
  Vxx_cyl_fill_mdl_ovlp_mass_bifuel : Inport  Port=33  Interpolate=off
  Sched10ms_ASXX_MWIN_FLW_filupxxxxg : TriggerPort  TriggerType=function-call  VariantControl=Variant
  A_Parabolic_model : Subsystem
  B_Optional_air_filling_estimation : Subsystem
  C_consolidation : Subsystem
  Cbx_vvtc_alti_cor_map_cfm : Constant  Value=Cbx_cyl_fill_efy_opt_cho
  DocBlock : Subsystem  mask(DocBlock){ECoderFlag=, DocumentType=Text}
      mask prompts: ECoderFlag "Simulink:blocks:docblockEmbeddedCoderFlagLabel"; DocumentType "Simulink:blocks:docblockDocTypeLabel"
      mask help: Use this block to save long descriptive text with the model. Double-clicking the block will open an editor.
      mask TypeOptions DocumentType: Text | RTF | HTML
      mask Display:
      | plot([.8 0 0 1 1 .8 .8 1],[1 1 0 0 .8 1 .8 .8]);
      | text(.5,.6,'DOC','horizontalalignment','center');
      | text(.95,.05,get_param(gcb,'DocumentType'),'verticalalignment','bottom','horizontalalignment','right');
  Switch1 : Switch  Criteria=u2 ~= 0  RndMeth=Zero  SaturateOnIntegerOverflow=on  InputSameDT=on
      settings: AttributesFormatString=Criteria=%<Criteria>
  Vxx_cyl_fill_efy : Outport  InitialOutput=1
      settings: AttributesFormatString=<initial=%<InitialOutput>>\n<whendisabled=%<OutputWhenDisabled>>
  Vxx_cyl_fill_efy_fil : Outport  Port=2  InitialOutput=1
      settings: AttributesFormatString=<initial=%<InitialOutput>>\n<whendisabled=%<OutputWhenDisabled>>
  Vxx_cyl_fill_efy_intk_mfld_prs_atm_prs_cor : Outport  Port=3  InitialOutput=101.3
      settings: AttributesFormatString=<initial=%<InitialOutput>>\n<whendisabled=%<OutputWhenDisabled>>
  Vxx_cyl_fill_efy_sp : Outport  Port=4  InitialOutput=1
      settings: AttributesFormatString=<initial=%<InitialOutput>>\n<whendisabled=%<OutputWhenDisabled>>
  Vxx_cyl_fill_efy_fil_sp : Outport  Port=5  InitialOutput=1
      settings: AttributesFormatString=<initial=%<InitialOutput>>\n<whendisabled=%<OutputWhenDisabled>>
  Vxx_cyl_igr_mass : Outport  Port=6  InitialOutput=0
      settings: AttributesFormatString=<initial=%<InitialOutput>>\n<whendisabled=%<OutputWhenDisabled>>
  Vxx_eng_vol_fill_efy : Outport  Port=7  InitialOutput=1
      settings: AttributesFormatString=<initial=%<InitialOutput>>\n<whendisabled=%<OutputWhenDisabled>>
  Vxx_eng_vol_fill_efy_fil : Outport  Port=8  InitialOutput=1
      settings: AttributesFormatString=<initial=%<InitialOutput>>\n<whendisabled=%<OutputWhenDisabled>>
  Vxx_cyl_fill_trap_efy_opt : Outport  Port=9  InitialOutput=1
      settings: AttributesFormatString=<initial=%<InitialOutput>>\n<whendisabled=%<OutputWhenDisabled>>
  Vxx_cyl_fill_mdl_intk_mfld_prs_diff_cor : Outport  Port=10  InitialOutput=0
      settings: AttributesFormatString=<initial=%<InitialOutput>>\n<whendisabled=%<OutputWhenDisabled>>
  Vxx_cyl_fill_mdl_ex_mfld_prs_rat_cor : Outport  Port=11  InitialOutput=1
      settings: AttributesFormatString=<initial=%<InitialOutput>>\n<whendisabled=%<OutputWhenDisabled>>
  wires:
  Cbx_vvtc_alti_cor_map_cfm/1 -> Switch1/2
  Vxx_vvt_ex_angl_cls/1 -> B_Optional_air_filling_estimation/2(Vxx_vvt_ex_angl_cls)  "Vxx_vvt_ex_angl_cls"
  Vxx_vvt_intk_angl_cls_l_lift/1 -> B_Optional_air_filling_estimation/3(Vxx_vvt_intk_angl_cls_l_lift)  "Vxx_vvt_intk_angl_cls_l_lift"
  Vxx_vvt_intk_angl_cls/1 -> B_Optional_air_filling_estimation/1(Vxx_vvt_intk_angl_cls)  "Vxx_vvt_intk_angl_cls"
  Vxx_vvt_ex_angl/1 -> B_Optional_air_filling_estimation/4(Vxx_vvt_ex_angl)  "Vxx_vvt_ex_angl"
  Vxx_avg_eng_spd/1 -> A_Parabolic_model/2(Vxx_avg_eng_spd), B_Optional_air_filling_estimation/7(Vxx_avg_eng_spd)  "Vxx_avg_eng_spd"
  Vxx_intk_mfld_prs/1 -> B_Optional_air_filling_estimation/6(Vxx_intk_mfld_prs), A_Parabolic_model/3(Vxx_intk_mfld_prs)  "Vxx_intk_mfld_prs"
  Vxx_vvt_intk_angl/1 -> B_Optional_air_filling_estimation/5(Vxx_vvt_intk_angl), A_Parabolic_model/4(Vxx_vvt_intk_angl)  "Vxx_vvt_intk_angl"
  Vxx_tq_fuel_typ_rat/1 -> B_Optional_air_filling_estimation/14(Vxx_tq_fuel_typ_rat), A_Parabolic_model/6(Vxx_tq_fuel_typ_rat)  "Vxx_tq_fuel_typ_rat"
  Vxx_intk_vlv_temp/1 -> A_Parabolic_model/1(Vxx_intk_vlv_temp), B_Optional_air_filling_estimation/8(Vxx_intk_vlv_temp)  "Vxx_intk_vlv_temp"
  Vxx_cyl_fill_efy_bas_bifuel/1 -> A_Parabolic_model/7(Vxx_cyl_fill_efy_bas_bifuel)  "Vxx_cyl_fill_efy_bas_bifuel"
  Vxx_cyl_fill_efy_temp_cor_bifuel/1 -> A_Parabolic_model/8(Vxx_cyl_fill_efy_temp_cor_bifuel)  "Vxx_cyl_fill_efy_temp_cor_bifuel"
  Vxx_eng_cool_temp/1 -> A_Parabolic_model/19(Vxx_eng_cool_temp)  "Vxx_eng_cool_temp"
  Vnx_eng_1st_sta_stt/1 -> A_Parabolic_model/20(Vnx_eng_1st_sta_stt)  "Vnx_eng_1st_sta_stt"
  Vxx_atm_prs/1 -> A_Parabolic_model/5(Vxx_atm_prs), B_Optional_air_filling_estimation/10(Vxx_atm_prs)  "Vxx_atm_prs"
  Vxx_cyl_fill_efy_vvt_intk_ex_cor/1 -> A_Parabolic_model/9(Vxx_cyl_fill_efy_vvt_intk_ex_cor)  "Vxx_cyl_fill_efy_vvt_intk_ex_cor"
  Vbx_aj_accel_decl/1 -> A_Parabolic_model/18(Vbx_aj_accel_decl)  "Vbx_aj_accel_decl"
  Vxx_cyl_fill_efy_dyn_cor_accel_t_cst_bifuel/1 -> A_Parabolic_model/10(Vxx_cyl_fill_efy_dyn_cor_accel_t_cst_bifuel)  "Vxx_cyl_fill_efy_dyn_cor_accel_t_cst_bifuel"
  Vxx_cyl_fill_efy_dyn_cor_thrml_bifuel/1 -> A_Parabolic_model/11(Vxx_cyl_fill_efy_dyn_cor_thrml_bifuel)  "Vxx_cyl_fill_efy_dyn_cor_thrml_bifuel"
  Vxx_cyl_fill_efy_dyn_cor_atm_prs_bifuel/1 -> A_Parabolic_model/12(Vxx_cyl_fill_efy_dyn_cor_atm_prs_bifuel)  "Vxx_cyl_fill_efy_dyn_cor_atm_prs_bifuel"
  Vxx_cyl_fill_efy_dyn_l_fill_fac_bifuel/1 -> A_Parabolic_model/15(Vxx_cyl_fill_efy_dyn_l_fill_fac_bifuel)  "Vxx_cyl_fill_efy_dyn_l_fill_fac_bifuel"
  Vxx_cyl_fill_efy_dyn_cor_cool_temp_bifuel/1 -> A_Parabolic_model/16(Vxx_cyl_fill_efy_dyn_cor_cool_temp_bifuel)  "Vxx_cyl_fill_efy_dyn_cor_cool_temp_bifuel"
  Vxx_cyl_fill_efy_dyn_cor_decl_t_cst_bifuel/1 -> A_Parabolic_model/17(Vxx_cyl_fill_efy_dyn_cor_decl_t_cst_bifuel)  "Vxx_cyl_fill_efy_dyn_cor_decl_t_cst_bifuel"
  Vxx_cyl_fill_efy_vvt_intk_cor_fac_1_bifuel/1 -> A_Parabolic_model/13(Vxx_cyl_fill_efy_vvt_intk_cor_fac_1_bifuel)  "Vxx_cyl_fill_efy_vvt_intk_cor_fac_1_bifuel"
  Vxx_cyl_fill_efy_vvt_intk_cor_fac_2_bifuel/1 -> A_Parabolic_model/14(Vxx_cyl_fill_efy_vvt_intk_cor_fac_2_bifuel)  "Vxx_cyl_fill_efy_vvt_intk_cor_fac_2_bifuel"
  A_Parabolic_model/4(Vxx_cyl_fill_efy_intk_mfld_prs_atm_prs_cor) -> Vxx_cyl_fill_efy_intk_mfld_prs_atm_prs_cor/1
  A_Parabolic_model/3(Vxt_cyl_fill_efy_para_mdl) -> Switch1/3
  Switch1/1 -> C_consolidation/5(Vxt_cyl_fill_efy)  "Vxt_cyl_fill_efy"
  Vxx_vvl_intk_l_lift_rat/1 -> C_consolidation/3(Vxx_vvl_intk_l_lift_rat)  "Vxx_vvl_intk_l_lift_rat"
  Vxx_vvl_intk_l_lift_rat_sp/1 -> C_consolidation/4(Vxx_vvl_intk_l_lift_rat_sp)  "Vxx_vvl_intk_l_lift_rat_sp"
  B_Optional_air_filling_estimation/1(Vxt_cyl_igr_mass) -> C_consolidation/1(Vxt_cyl_igr_mass)
  B_Optional_air_filling_estimation/2(Vxt_cyl_fill_trap_efy_opt) -> C_consolidation/2(Vxt_cyl_fill_trap_efy_opt)
  C_consolidation/1(Vxx_cyl_fill_efy) -> Vxx_cyl_fill_efy/1
  C_consolidation/2(Vxx_cyl_fill_efy_fil) -> Vxx_cyl_fill_efy_fil/1
  C_consolidation/3(Vxx_cyl_fill_efy_sp) -> Vxx_cyl_fill_efy_sp/1
  C_consolidation/4(Vxx_cyl_fill_efy_fil_sp) -> Vxx_cyl_fill_efy_fil_sp/1
  C_consolidation/5(Vxx_cyl_igr_mass) -> Vxx_cyl_igr_mass/1
  C_consolidation/6(Vxx_eng_vol_fill_efy) -> Vxx_eng_vol_fill_efy/1
  C_consolidation/7(Vxx_eng_vol_fill_efy_fil) -> Vxx_eng_vol_fill_efy_fil/1
  C_consolidation/8(Vxx_cyl_fill_trap_efy_opt) -> Vxx_cyl_fill_trap_efy_opt/1
  Vxx_ex_mfld_temp/1 -> B_Optional_air_filling_estimation/9(Vxx_ex_mfld_temp)  "Vxx_ex_mfld_temp"
  Vxx_pft_rel_diff_prs/1 -> B_Optional_air_filling_estimation/11(Vxx_pft_rel_diff_prs)  "Vxx_pft_rel_diff_prs"
  Vxx_ex_mfld_prs/1 -> B_Optional_air_filling_estimation/12(Vxx_ex_mfld_prs)  "Vxx_ex_mfld_prs"
  Vxx_mdl_ref_ex_mfld_prs/1 -> B_Optional_air_filling_estimation/13(Vxx_mdl_ref_ex_mfld_prs)  "Vxx_mdl_ref_ex_mfld_prs"
  B_Optional_air_filling_estimation/3(Vxt_cyl_fill_efy_opt) -> Switch1/1
  Vxx_cyl_fill_mdl_pump_mass_bas_bifuel/1 -> B_Optional_air_filling_estimation/15(Vxx_cyl_fill_mdl_pump_mass_bas_bifuel)  "Vxx_cyl_fill_mdl_pump_mass_bas_bifuel"
  Vxx_cyl_fill_mdl_ovlp_mass_bifuel/1 -> B_Optional_air_filling_estimation/16(Vxx_cyl_fill_mdl_ovlp_mass_bifuel)  "Vxx_cyl_fill_mdl_ovlp_mass_bifuel"
  Vxx_cyl_igr_mass_bifuel/1 -> B_Optional_air_filling_estimation/17(Vxx_cyl_igr_mass_bifuel)  "Vxx_cyl_igr_mass_bifuel"
  A_Parabolic_model/2(Vxx_cyl_fill_efy_dyn_cor) -> B_Optional_air_filling_estimation/19(Vxx_cyl_fill_efy_dyn_cor)
  A_Parabolic_model/1(Vxx_cyl_fill_efy_temp_cor) -> B_Optional_air_filling_estimation/18(Vxx_cyl_fill_efy_temp_cor)
  B_Optional_air_filling_estimation/5(Vxx_cyl_fill_mdl_ex_mfld_prs_rat_cor) -> Vxx_cyl_fill_mdl_ex_mfld_prs_rat_cor/1
  B_Optional_air_filling_estimation/4(Vxx_cyl_fill_mdl_intk_mfld_prs_diff_cor) -> Vxx_cyl_fill_mdl_intk_mfld_prs_diff_cor/1

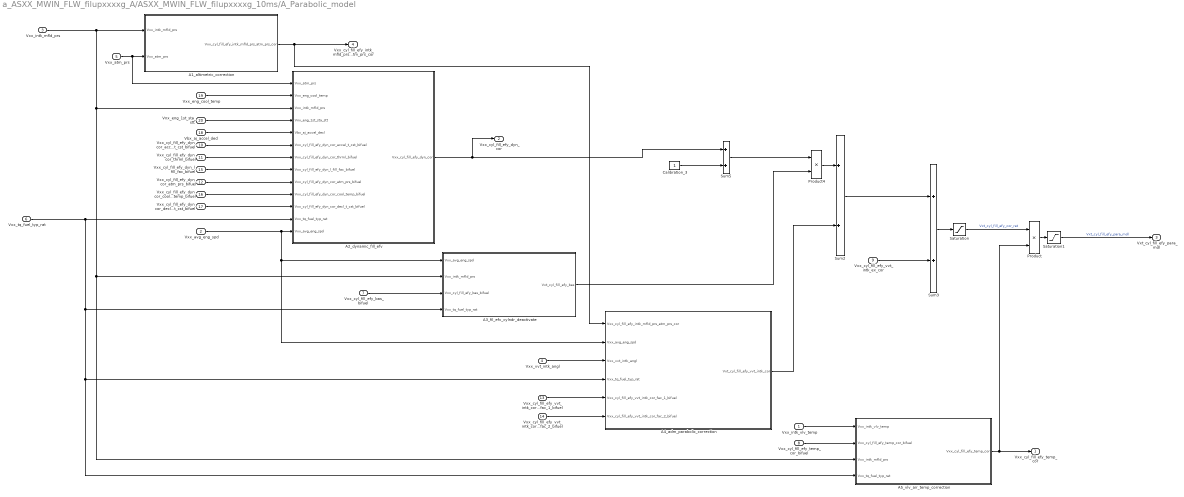
== system a_ASXX_MWIN_FLW_filupxxxxg_A/ASXX_MWIN_FLW_filupxxxxg_10ms/A_Parabolic_model ==
  Vxx_intk_vlv_temp : Inport  Interpolate=off
  Vxx_avg_eng_spd : Inport  Port=2  Interpolate=off
  Vxx_intk_mfld_prs : Inport  Port=3  Interpolate=off
  Vxx_vvt_intk_angl : Inport  Port=4  Interpolate=off
  Vxx_atm_prs : Inport  Port=5  Interpolate=off
  Vxx_tq_fuel_typ_rat : Inport  Port=6  Interpolate=off
  Vxx_cyl_fill_efy_bas_bifuel : Inport  Port=7  Interpolate=off
  Vxx_cyl_fill_efy_temp_cor_bifuel : Inport  Port=8  Interpolate=off
  Vxx_cyl_fill_efy_vvt_intk_ex_cor : Inport  Port=9  Interpolate=off
  Vxx_cyl_fill_efy_dyn_cor_accel_t_cst_bifuel : Inport  Port=10  Interpolate=off
  Vxx_cyl_fill_efy_dyn_cor_thrml_bifuel : Inport  Port=11  Interpolate=off
  Vxx_cyl_fill_efy_dyn_cor_atm_prs_bifuel : Inport  Port=12  Interpolate=off
  Vxx_cyl_fill_efy_vvt_intk_cor_fac_1_bifuel : Inport  Port=13  Interpolate=off
  Vxx_cyl_fill_efy_vvt_intk_cor_fac_2_bifuel : Inport  Port=14  Interpolate=off
  Vxx_cyl_fill_efy_dyn_l_fill_fac_bifuel : Inport  Port=15  Interpolate=off
  Vxx_cyl_fill_efy_dyn_cor_cool_temp_bifuel : Inport  Port=16  Interpolate=off
  Vxx_cyl_fill_efy_dyn_cor_decl_t_cst_bifuel : Inport  Port=17  Interpolate=off
  Vbx_aj_accel_decl : Inport  Port=18  Interpolate=off
  Vxx_eng_cool_temp : Inport  Port=19  Interpolate=off
  Vnx_eng_1st_sta_stt : Inport  Port=20  Interpolate=off
  A1_altimetric_correction : Subsystem
  A2_dynamic_fill_efv : Subsystem
  A3_fil_efv_cylndr_deactivate : Subsystem
  A4_adm_parabolic_correction : Subsystem
  A5_vlv_air_temp_correction : Subsystem
  Calibration_3 : Constant  OutDataTypeStr=single
  Product : Product  Inputs=**  OutDataTypeStr=Inherit: Inherit via back propagation  RndMeth=Zero
  Product4 : Product  Inputs=**  OutDataTypeStr=Inherit: Inherit via back propagation  RndMeth=Zero
  Saturation : Saturate  UpperLimit=2  LowerLimit=0  RndMeth=Zero
      settings: AttributesFormatString=<limits=%<UpperLimit>/%<LowerLimit>>
  Saturation1 : Saturate  UpperLimit=2  LowerLimit=0  RndMeth=Zero
      settings: AttributesFormatString=<limits=%<UpperLimit>/%<LowerLimit>>
  Sum2 : Sum  OutDataTypeStr=Inherit: Inherit via back propagation  RndMeth=Zero  InputSameDT=on
  Sum3 : Sum  OutDataTypeStr=Inherit: Inherit via back propagation  RndMeth=Zero  InputSameDT=on
  Sum5 : Sum  OutDataTypeStr=Inherit: Inherit via back propagation  RndMeth=Zero  InputSameDT=on
  Vxx_cyl_fill_efy_temp_cor : Outport
  Vxx_cyl_fill_efy_dyn_cor : Outport  Port=2
  Vxt_cyl_fill_efy_para_mdl : Outport  Port=3
  Vxx_cyl_fill_efy_intk_mfld_prs_atm_prs_cor : Outport  Port=4
  wires:
  Vxx_cyl_fill_efy_dyn_cor_accel_t_cst_bifuel/1 -> A2_dynamic_fill_efv/6(Vxx_cyl_fill_efy_dyn_cor_accel_t_cst_bifuel)
  Vxx_vvt_intk_angl/1 -> A4_adm_parabolic_correction/3(Vxx_vvt_intk_angl)
  Vxx_intk_vlv_temp/1 -> A5_vlv_air_temp_correction/1(Vxx_intk_vlv_temp)
  Vxx_cyl_fill_efy_temp_cor_bifuel/1 -> A5_vlv_air_temp_correction/2(Vxx_cyl_fill_efy_temp_cor_bifuel)
  Vxx_eng_cool_temp/1 -> A2_dynamic_fill_efv/2(Vxx_eng_cool_temp)
  Vnx_eng_1st_sta_stt/1 -> A2_dynamic_fill_efv/4(Vnx_eng_1st_sta_stt)
  Vxx_cyl_fill_efy_bas_bifuel/1 -> A3_fil_efv_cylndr_deactivate/3(Vxx_cyl_fill_efy_bas_bifuel)
  Vxx_cyl_fill_efy_vvt_intk_ex_cor/1 -> Sum3/2
  Vbx_aj_accel_decl/1 -> A2_dynamic_fill_efv/5(Vbx_aj_accel_decl)
  A4_adm_parabolic_correction/1(Vxt_cyl_fill_efy_vvt_intk_cor) -> Sum2/2
  Product4/1 -> Sum2/1
  Vxx_cyl_fill_efy_vvt_intk_cor_fac_2_bifuel/1 -> A4_adm_parabolic_correction/6(Vxx_cyl_fill_efy_vvt_intk_cor_fac_2_bifuel)
  Vxx_intk_mfld_prs/1 -> A5_vlv_air_temp_correction/3(Vxx_intk_mfld_prs), A3_fil_efv_cylndr_deactivate/2(Vxx_intk_mfld_prs), A2_dynamic_fill_efv/3(Vxx_intk_mfld_prs), A1_altimetric_correction/1(Vxx_intk_mfld_prs)
  Saturation/1 -> Product/1  "Vxt_cyl_fill_efy_cor_rat"
  Sum3/1 -> Saturation/1
  Vxx_atm_prs/1 -> A1_altimetric_correction/2(Vxx_atm_prs), A2_dynamic_fill_efv/1(Vxx_atm_prs)
  A3_fil_efv_cylndr_deactivate/1(Vxt_cyl_fill_efy_bas) -> Product4/2
  Vxx_avg_eng_spd/1 -> A3_fil_efv_cylndr_deactivate/1(Vxx_avg_eng_spd), A4_adm_parabolic_correction/2(Vxx_avg_eng_spd), A2_dynamic_fill_efv/13(Vxx_avg_eng_spd)
  Sum2/1 -> Sum3/1
  A2_dynamic_fill_efv/1(Vxx_cyl_fill_efy_dyn_cor) -> Vxx_cyl_fill_efy_dyn_cor/1, Sum5/1
  Vxx_cyl_fill_efy_vvt_intk_cor_fac_1_bifuel/1 -> A4_adm_parabolic_correction/5(Vxx_cyl_fill_efy_vvt_intk_cor_fac_1_bifuel)
  Vxx_cyl_fill_efy_dyn_cor_decl_t_cst_bifuel/1 -> A2_dynamic_fill_efv/11(Vxx_cyl_fill_efy_dyn_cor_decl_t_cst_bifuel)
  Vxx_cyl_fill_efy_dyn_cor_cool_temp_bifuel/1 -> A2_dynamic_fill_efv/10(Vxx_cyl_fill_efy_dyn_cor_cool_temp_bifuel)
  Vxx_cyl_fill_efy_dyn_l_fill_fac_bifuel/1 -> A2_dynamic_fill_efv/8(Vxx_cyl_fill_efy_dyn_l_fill_fac_bifuel)
  Vxx_tq_fuel_typ_rat/1 -> A5_vlv_air_temp_correction/4(Vxx_tq_fuel_typ_rat), A4_adm_parabolic_correction/4(Vxx_tq_fuel_typ_rat), A3_fil_efv_cylndr_deactivate/4(Vxx_tq_fuel_typ_rat), A2_dynamic_fill_efv/12(Vxx_tq_fuel_typ_rat)
  A5_vlv_air_temp_correction/1(Vxx_cyl_fill_efy_temp_cor) -> Vxx_cyl_fill_efy_temp_cor/1, Product/2
  Vxx_cyl_fill_efy_dyn_cor_atm_prs_bifuel/1 -> A2_dynamic_fill_efv/9(Vxx_cyl_fill_efy_dyn_cor_atm_prs_bifuel)
  Vxx_cyl_fill_efy_dyn_cor_thrml_bifuel/1 -> A2_dynamic_fill_efv/7(Vxx_cyl_fill_efy_dyn_cor_thrml_bifuel)
  A1_altimetric_correction/1(Vxx_cyl_fill_efy_intk_mfld_prs_atm_prs_cor) -> Vxx_cyl_fill_efy_intk_mfld_prs_atm_prs_cor/1, A4_adm_parabolic_correction/1(Vxx_cyl_fill_efy_intk_mfld_prs_atm_prs_cor)
  Product/1 -> Saturation1/1
  Saturation1/1 -> Vxt_cyl_fill_efy_para_mdl/1  "Vxt_cyl_fill_efy_para_mdl"
  Calibration_3/1 -> Sum5/2
  Sum5/1 -> Product4/1

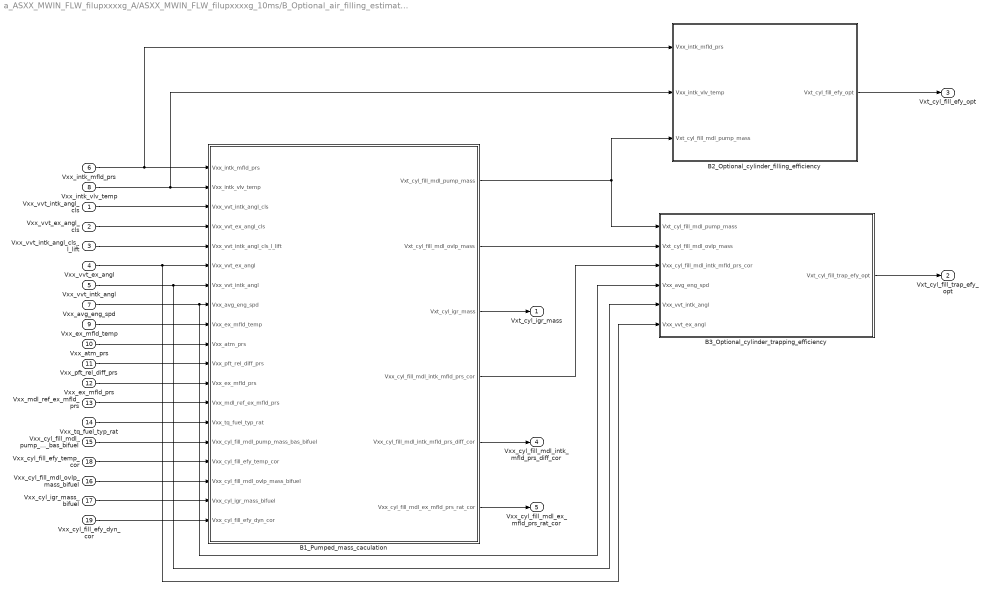
== system a_ASXX_MWIN_FLW_filupxxxxg_A/ASXX_MWIN_FLW_filupxxxxg_10ms/B_Optional_air_filling_estimation ==
  Vxx_vvt_intk_angl_cls : Inport  Interpolate=off
  Vxx_vvt_ex_angl_cls : Inport  Port=2  Interpolate=off
  Vxx_vvt_intk_angl_cls_l_lift : Inport  Port=3  Interpolate=off
  Vxx_vvt_ex_angl : Inport  Port=4  Interpolate=off
  Vxx_vvt_intk_angl : Inport  Port=5  Interpolate=off
  Vxx_intk_mfld_prs : Inport  Port=6  Interpolate=off
  Vxx_avg_eng_spd : Inport  Port=7  Interpolate=off
  Vxx_intk_vlv_temp : Inport  Port=8  Interpolate=off
  Vxx_ex_mfld_temp : Inport  Port=9  Interpolate=off
  Vxx_atm_prs : Inport  Port=10  Interpolate=off
  Vxx_pft_rel_diff_prs : Inport  Port=11  Interpolate=off
  Vxx_ex_mfld_prs : Inport  Port=12  Interpolate=off
  Vxx_mdl_ref_ex_mfld_prs : Inport  Port=13  Interpolate=off
  Vxx_tq_fuel_typ_rat : Inport  Port=14  Interpolate=off
  Vxx_cyl_fill_mdl_pump_mass_bas_bifuel : Inport  Port=15  Interpolate=off
  Vxx_cyl_fill_mdl_ovlp_mass_bifuel : Inport  Port=16  Interpolate=off
  Vxx_cyl_igr_mass_bifuel : Inport  Port=17  Interpolate=off
  Vxx_cyl_fill_efy_temp_cor : Inport  Port=18  Interpolate=off
  Vxx_cyl_fill_efy_dyn_cor : Inport  Port=19  Interpolate=off
  B1_Pumped_mass_caculation : Subsystem
  B2_Optional_cylinder_filling_efficiency : Subsystem
  B3_Optional_cylinder_trapping_efficiency : Subsystem
  Vxt_cyl_igr_mass : Outport
  Vxt_cyl_fill_trap_efy_opt : Outport  Port=2
  Vxt_cyl_fill_efy_opt : Outport  Port=3
  Vxx_cyl_fill_mdl_intk_mfld_prs_diff_cor : Outport  Port=4
  Vxx_cyl_fill_mdl_ex_mfld_prs_rat_cor : Outport  Port=5
  wires:
  B3_Optional_cylinder_trapping_efficiency/1(Vxt_cyl_fill_trap_efy_opt) -> Vxt_cyl_fill_trap_efy_opt/1
  Vxx_vvt_intk_angl_cls/1 -> B1_Pumped_mass_caculation/3(Vxx_vvt_intk_angl_cls)
  Vxx_vvt_ex_angl_cls/1 -> B1_Pumped_mass_caculation/4(Vxx_vvt_ex_angl_cls)
  Vxx_vvt_intk_angl_cls_l_lift/1 -> B1_Pumped_mass_caculation/5(Vxx_vvt_intk_angl_cls_l_lift)
  Vxx_vvt_intk_angl/1 -> B3_Optional_cylinder_trapping_efficiency/5(Vxx_vvt_intk_angl), B1_Pumped_mass_caculation/7(Vxx_vvt_intk_angl)
  Vxx_intk_mfld_prs/1 -> B1_Pumped_mass_caculation/1(Vxx_intk_mfld_prs), B2_Optional_cylinder_filling_efficiency/1(Vxx_intk_mfld_prs)
  Vxx_avg_eng_spd/1 -> B3_Optional_cylinder_trapping_efficiency/4(Vxx_avg_eng_spd), B1_Pumped_mass_caculation/8(Vxx_avg_eng_spd)
  Vxx_intk_vlv_temp/1 -> B1_Pumped_mass_caculation/2(Vxx_intk_vlv_temp), B2_Optional_cylinder_filling_efficiency/2(Vxx_intk_vlv_temp)
  Vxx_ex_mfld_temp/1 -> B1_Pumped_mass_caculation/9(Vxx_ex_mfld_temp)
  Vxx_atm_prs/1 -> B1_Pumped_mass_caculation/10(Vxx_atm_prs)
  Vxx_pft_rel_diff_prs/1 -> B1_Pumped_mass_caculation/11(Vxx_pft_rel_diff_prs)
  Vxx_ex_mfld_prs/1 -> B1_Pumped_mass_caculation/12(Vxx_ex_mfld_prs)
  Vxx_mdl_ref_ex_mfld_prs/1 -> B1_Pumped_mass_caculation/13(Vxx_mdl_ref_ex_mfld_prs)
  B1_Pumped_mass_caculation/1(Vxt_cyl_fill_mdl_pump_mass) -> B3_Optional_cylinder_trapping_efficiency/1(Vxt_cyl_fill_mdl_pump_mass), B2_Optional_cylinder_filling_efficiency/3(Vxt_cyl_fill_mdl_pump_mass)
  B2_Optional_cylinder_filling_efficiency/1(Vxt_cyl_fill_efy_opt) -> Vxt_cyl_fill_efy_opt/1
  B1_Pumped_mass_caculation/2(Vxt_cyl_fill_mdl_ovlp_mass) -> B3_Optional_cylinder_trapping_efficiency/2(Vxt_cyl_fill_mdl_ovlp_mass)
  Vxx_tq_fuel_typ_rat/1 -> B1_Pumped_mass_caculation/14(Vxx_tq_fuel_typ_rat)
  Vxx_cyl_fill_mdl_pump_mass_bas_bifuel/1 -> B1_Pumped_mass_caculation/15(Vxx_cyl_fill_mdl_pump_mass_bas_bifuel)
  Vxx_cyl_fill_efy_dyn_cor/1 -> B1_Pumped_mass_caculation/19(Vxx_cyl_fill_efy_dyn_cor)
  Vxx_cyl_fill_efy_temp_cor/1 -> B1_Pumped_mass_caculation/16(Vxx_cyl_fill_efy_temp_cor)
  B1_Pumped_mass_caculation/3(Vxt_cyl_igr_mass) -> Vxt_cyl_igr_mass/1
  Vxx_cyl_fill_mdl_ovlp_mass_bifuel/1 -> B1_Pumped_mass_caculation/17(Vxx_cyl_fill_mdl_ovlp_mass_bifuel)
  Vxx_cyl_igr_mass_bifuel/1 -> B1_Pumped_mass_caculation/18(Vxx_cyl_igr_mass_bifuel)
  Vxx_vvt_ex_angl/1 -> B3_Optional_cylinder_trapping_efficiency/6(Vxx_vvt_ex_angl), B1_Pumped_mass_caculation/6(Vxx_vvt_ex_angl)
  B1_Pumped_mass_caculation/4(Vxx_cyl_fill_mdl_intk_mfld_prs_cor) -> B3_Optional_cylinder_trapping_efficiency/3(Vxx_cyl_fill_mdl_intk_mfld_prs_cor)
  B1_Pumped_mass_caculation/6(Vxx_cyl_fill_mdl_ex_mfld_prs_rat_cor) -> Vxx_cyl_fill_mdl_ex_mfld_prs_rat_cor/1
  B1_Pumped_mass_caculation/5(Vxx_cyl_fill_mdl_intk_mfld_prs_diff_cor) -> Vxx_cyl_fill_mdl_intk_mfld_prs_diff_cor/1
